simulink model "Ejercicio11_8_sim"  (R2023b)
settings: Solver=VariableStepAuto  StartTime=0.0  StopTime=10.0  MaxStep=1e-5  RelTol=1e-3
values from neighbouring files (symbols this model uses):
  b = 1    [Ejercicio11_8.m]    (also in Ejercicio25_8.m)
  Jm = 1    [Ejercicio11_8.m]    (also in Ejercicio25_8.m)
  kl = 0.5    [Ejercicio11_8.m]    (also in Ejercicio25_8.m)
  km = 1    [Ejercicio11_8.m]    (also in Ejercicio25_8.m)
  Tm = 1    [Ejercicio11_8.m]    (also in Ejercicio25_8.m)
undefined symbols (not defined in the file or in its folder): magnitude
settings Model: Creator=tomas  LastModifiedBy=tomas

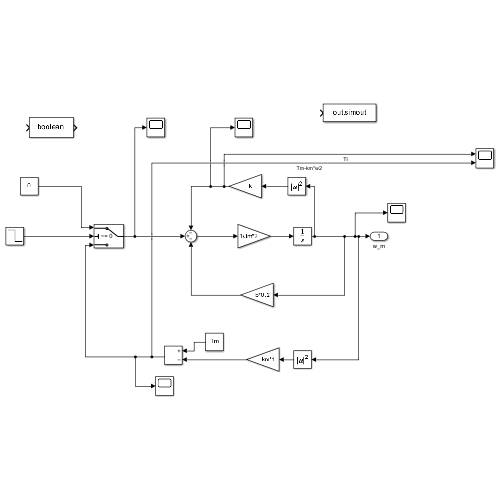
[thumbnail: Simulink's stored preview of the top-level diagram]
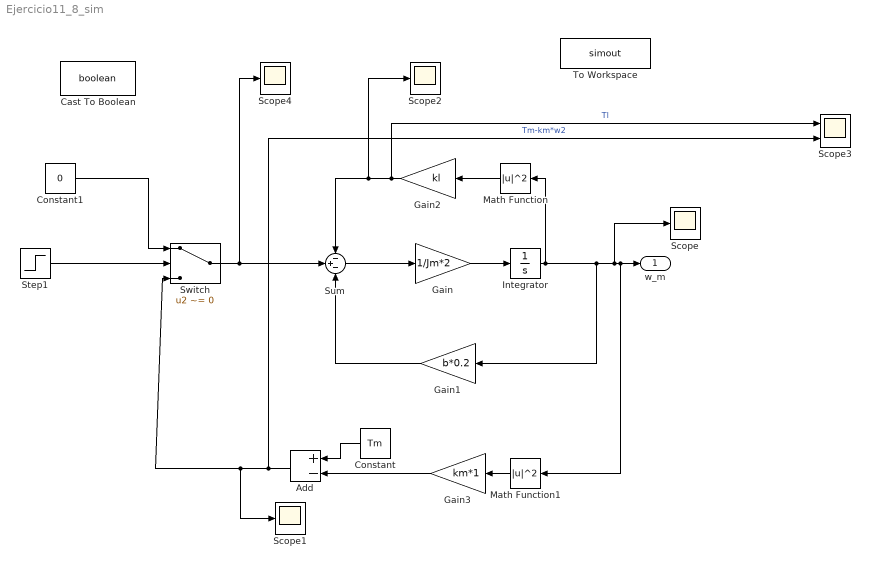
== system Ejercicio11_8_sim ==
  Add : Sum  Inputs=+-
  Cast To Boolean : DataTypeConversion  OutDataTypeStr=boolean  SaturateOnIntegerOverflow=off  RndMeth=Floor
  Constant : Constant  Value=Tm
  Constant1 : Constant  Value=0
  Gain : Gain  Gain=1/Jm*2
  Gain1 : Gain  Gain=b*0.2
  Gain2 : Gain  Gain=kl
  Gain3 : Gain  Gain=km*1
  Integrator : Integrator
  Math Function : Math  Operator=magnitude^2
  Math Function1 : Math  Operator=magnitude^2
  Scope{,1..2,4} (4 alike) : Scope
  Scope3 : Scope  NumInputPorts=2
  Step1 : Step  Time=3  Before=1  After=0  SampleTime=0
  Sum : Sum  Inputs=-+-
  Switch : Switch  Criteria=u2 ~= 0  SaturateOnIntegerOverflow=off  InputSameDT=off
  To Workspace : ToWorkspace  VariableName=simout  SaveFormat=Timeseries  SampleTime=-1
  w_m : Outport
  wires:
  Gain/1 -> Integrator/1
  Sum/1 -> Gain/1
  Gain1/1 -> Sum/3
  Math Function/1 -> Gain2/1
  Gain2/1 -> Scope3/1, Scope2/1, Sum/1  "Tl"
  Switch/1 -> Scope4/1, Sum/2
  Math Function1/1 -> Gain3/1
  Gain3/1 -> Add/2
  Integrator/1 -> Math Function/1, Gain1/1, Scope/1, Math Function1/1, w_m/1
  Constant/1 -> Add/1
  Add/1 -> Scope3/2, Scope1/1, Switch/3  "Tm-km*w2"
  Constant1/1 -> Switch/1
  Step1/1 -> Switch/2
